simulink model "pi_control"  (R2023b)
settings: Solver=VariableStepAuto  StartTime=0.0  StopTime=30  RelTol=1e-3
model workspace (MAT data in the model file):
  Ki = Simulink.Parameter
  Ki.Value = 0
  Ki.DataType = 'auto'
  Ki.Complexity = 'real'
  Ki.Dimensions = [1 1]
  Kp = Simulink.Parameter
  Kp.Value = 0
  Kp.DataType = 'auto'
  Kp.Complexity = 'real'
  Kp.Dimensions = [1 1]
settings Model: Creator=kijun  LastModifiedBy=kijun

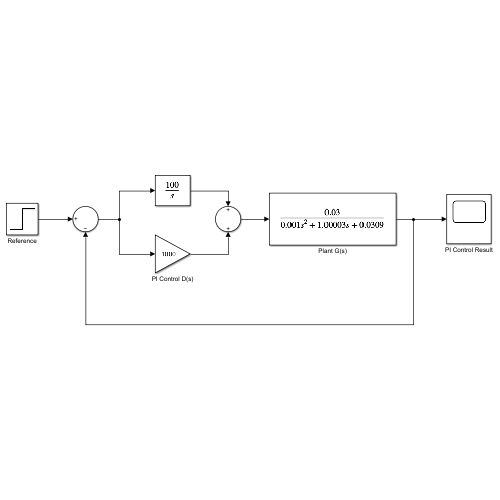
[thumbnail: Simulink's stored preview of the top-level diagram]
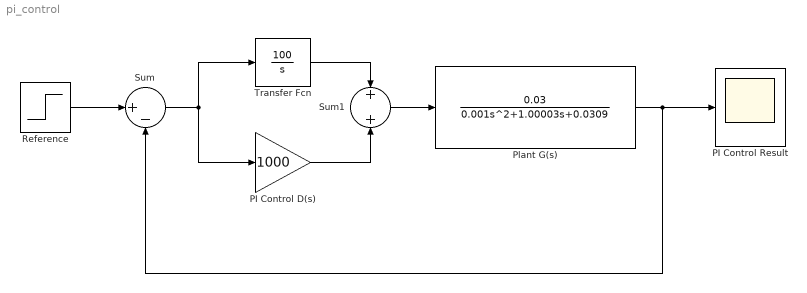
== system pi_control ==
  PI Control D(s) : Gain  Gain=1000
  PI Control Result : Scope
  Plant G(s) : TransferFcn  Numerator=[0.03]  Denominator=[0.001 1.00003 0.0309]
  Reference : Step  Time=0  SampleTime=0
  Sum : Sum  Inputs=|+-
  Sum1 : Sum  Inputs=+|+
  Transfer Fcn : TransferFcn  Numerator=100  Denominator=[1 0]
  wires:
  Sum1/1 -> Plant G(s)/1
  PI Control D(s)/1 -> Sum1/2
  Transfer Fcn/1 -> Sum1/1
  Plant G(s)/1 -> PI Control Result/1, Sum/2
  Sum/1 -> PI Control D(s)/1, Transfer Fcn/1
  Reference/1 -> Sum/1
